simulink library "TElib"  (Simulink 10.2)
settings: Solver=VariableStepAuto  StartTime=0.0  StopTime=10.0  RelTol=1e-3
undefined symbols (not defined in the file): Ts
libraries: $bdroot x1
settings Model: Creator=mazen  LastModifiedBy=mazen

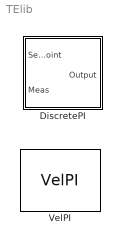
== system TElib ==
  DiscretePI : Subsystem  mask{Kc=0, Ti=inf, Ts=1, x0=0, Hi=1, Lo=-1}
  VelPI : $bdroot/DiscretePI/VelPI  Kc=Kc  Ti=Ti  Ts=Ts

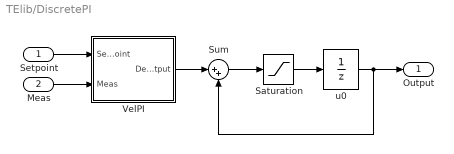
== system TElib/DiscretePI ==
  Setpoint : Inport
  Meas : Inport  Port=2
  Saturation : Saturate  UpperLimit=Hi  LowerLimit=Lo
  Sum : Sum  Inputs=|++  SaturateOnIntegerOverflow=on
  VelPI : Subsystem  mask{Kc=Kc, Ti=Ti, Ts=Ts}
  u0 : UnitDelay  InitialCondition=x0  SampleTime=Ts
  Output : Outport
  wires:
  Sum/1 -> Saturation/1
  VelPI/1(Delta Output) -> Sum/1
  Saturation/1 -> u0/1
  u0/1 -> Sum/2, Output/1
  Meas/1 -> VelPI/2(Meas)
  Setpoint/1 -> VelPI/1(Setpoint)

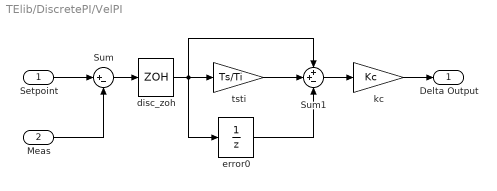
== system TElib/DiscretePI/VelPI ==
  Setpoint : Inport
  Meas : Inport  Port=2
  Sum : Sum  Inputs=|+-  SaturateOnIntegerOverflow=on
  Sum1 : Sum  Inputs=++-  SaturateOnIntegerOverflow=on
  disc_zoh : ZeroOrderHold  SampleTime=Ts
  error0 : UnitDelay  SampleTime=Ts
  kc : Gain  Gain=Kc  SaturateOnIntegerOverflow=on  OutDataTypeStr=Inherit: Same as input  ParamDataTypeStr=Inherit: Same as input
  tsti : Gain  Gain=Ts/Ti  SaturateOnIntegerOverflow=on  OutDataTypeStr=Inherit: Same as input  ParamDataTypeStr=Inherit: Same as input
  Delta Output : Outport
  wires:
  Setpoint/1 -> Sum/1
  Meas/1 -> Sum/2
  kc/1 -> Delta Output/1
  Sum1/1 -> kc/1
  tsti/1 -> Sum1/2
  error0/1 -> Sum1/3
  Sum/1 -> disc_zoh/1
  disc_zoh/1 -> tsti/1, error0/1, Sum1/1
